simulink model "komplementaryfilter_experiment"  (R2023a)
settings: Solver=FixedStepAuto  StartTime=0.0  StopTime=tend  FixedStep=0.02  RelTol=1e-3
libraries: cstblocks x2, dspsigops x2
settings Model: Creator=Xenjamo  LastModifiedBy=Xenjamo

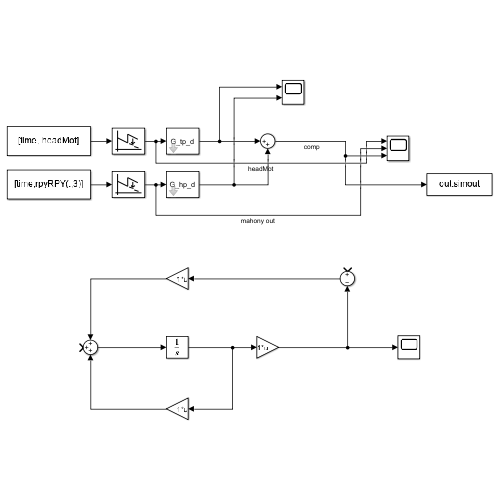
[thumbnail: Simulink's stored preview of the top-level diagram]
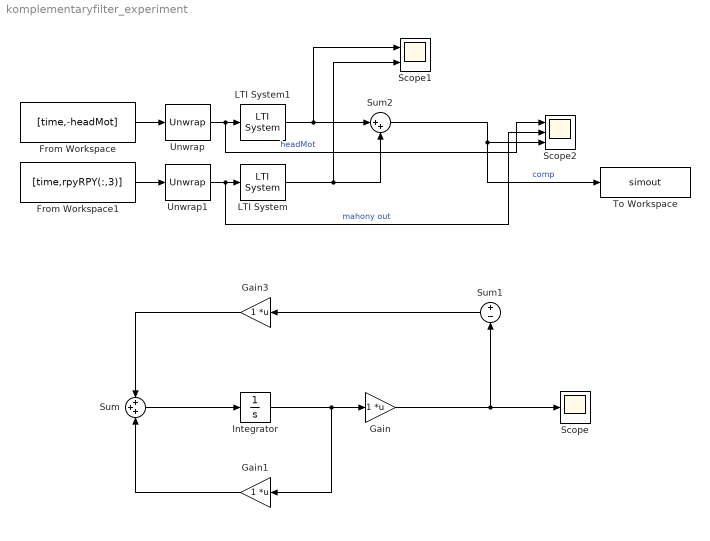
== system komplementaryfilter_experiment ==
  From Workspace : FromWorkspace  VariableName=[time,-headMot]
  From Workspace1 : FromWorkspace  VariableName=[time,rpyRPY(:,3)]
  Gain : Gain  Multiplication=Matrix(K*u)
  Gain1 : Gain  Multiplication=Matrix(K*u)
  Gain3 : Gain  Multiplication=Matrix(K*u)
  Integrator : Integrator
  LTI System : cstblocks/LTI System  sys=G_hp_d  IC=[]
  LTI System1 : cstblocks/LTI System  sys=G_tp_d  IC=[]
  Scope : Scope
  Scope1 : Scope  NumInputPorts=2
  Scope2 : Scope  NumInputPorts=3
  Sum : Sum  Inputs=+++
  Sum1 : Sum  Inputs=+|-
  Sum2 : Sum  Inputs=|++
  To Workspace : ToWorkspace  VariableName=simout  SaveFormat=Timeseries  SampleTime=-1
  Unwrap : dspsigops/Unwrap  tol=pi  InputProcessing=Columns as channels (frame based)  running=off
  Unwrap1 : dspsigops/Unwrap  tol=pi  InputProcessing=Columns as channels (frame based)  running=off
  wires:
  Sum/1 -> Integrator/1
  Integrator/1 -> Gain/1, Gain1/1
  Gain/1 -> Scope/1, Sum1/2
  Sum1/1 -> Gain3/1
  Gain1/1 -> Sum/3
  Gain3/1 -> Sum/1
  From Workspace1/1 -> Unwrap1/1
  From Workspace/1 -> Unwrap/1
  Unwrap/1 -> Scope2/1, LTI System1/1  "headMot"
  Unwrap1/1 -> Scope2/2, LTI System/1  "mahony out"
  LTI System/1 -> Sum2/2, Scope1/2
  LTI System1/1 -> Sum2/1, Scope1/1
  Sum2/1 -> To Workspace/1, Scope2/3  "comp"
